simulink model "control_3quads_attached_Kumar"  (R2019a)
settings: Solver=FixedStepAuto  StartTime=0.0  StopTime=10  FixedStep=0.025  RelTol=1e-3  EnableMultiTasking=on
InitFcn:
  | global clientID;
  | clientID=-1;
  | 
  | global R_t;
  | global A_t;
  | global P_t;
  | global H;
  | global Q;
  | global N;
  | 
  | R_t=eye(3);
  | A_t=eye(3)*0;
  | P_t=eye(3)*0.001;
  | H=eye(3);
  | Q=eye(3);
  | N=eye(3);
undefined symbols (not defined in the file or in its folder): Angular, Linear, sigbuilder_block
libraries: robotlib x7, dspindex x3, simulink x1
settings Model: Creator=Kleber Cabral  LastModifiedBy=Kleber Cabral
settings DataIOCC: SaveFormat=Array  ReturnWorkspaceOutputs=off
settings OptimizationCC: LifeSpan=inf
settings DebuggingCC: SolverPrmCheckMsg=warning  SFUnexpectedBacktrackingDiag=warning  SFNoUnconditionalDefaultTransitionDiag=warning  ArithmeticOperatorsInVariantConditions=warning
settings HardwareCC: ProdBitPerPointer=32  ProdBitPerSizeT=32  ProdBitPerPtrDiffT=32  ProdLargestAtomicFloat=None  ProdIntDivRoundTo=Undefined  ProdEndianess=Unspecified  ProdWordSize=32  ProdHWDeviceType=32-bit Generic
settings ModelReferenceCC: PropagateSignalLabelsOutOfModel=off
settings SFSimCC: SimUseLocalCustomCode=off
settings RTWCC: RTWUseLocalCustomCode=off
settings CodeAppCC: StateflowObjectComments=on
settings GRTTargetCC: TargetLangStandard=C89/C90 (ANSI)  GeneratePreprocessorConditionals=Disable all
settings ConfigComp: CovMetricSettings=dw  CovHtmlReporting=on  CovSaveCumulativeToWorkspaceVar=on  CovSaveSingleToWorkspaceVar=on  CovExternalEMLEnable=off  CovSFcnEnable=off

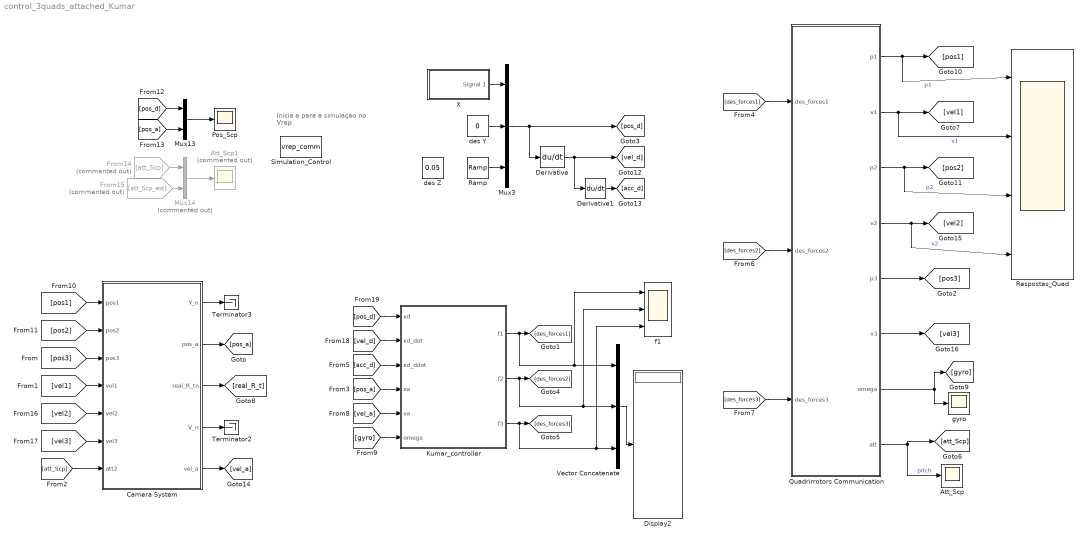
== system control_3quads_attached_Kumar ==
  note: Inicia e para a simulaçao no Vrep
  Att_Scp : Scope
  Att_Scp1 : Scope  Commented=on
  Camera System : Subsystem
  Derivative : Derivative
  Derivative1 : Derivative
  Display2 : Display
      settings: Decimation=3
  From14 : From  Commented=on  GotoTag=att_Scp
  From15 : From  Commented=on  GotoTag=att_Scp_est
  Kumar_controller : MATLAB Function  TreatAsAtomicUnit=on
  Mux13 : Mux  Inputs=2
  Mux14 : Mux  Commented=on  Inputs=2
  Mux3 : Mux  Inputs=3
  Pos_Scp : Scope
  Quadrirrotors Communication : Subsystem
  Ramp : simulink/Sources/Ramp  slope=0.05  start=1  InitialOutput=0
  Respostas_Quad : Scope  NumInputPorts=4
  Simulation_Control : S-Function  FunctionName=vrep_comm  SFunctionDeploymentMode=off  EnableBusSupport=off
  Terminator2 : Terminator
  Terminator3 : Terminator
  Vector Concatenate : Concatenate  NumInputs=3
  X : Subsystem  Tag=STV Subsys  LoadFcn=sigbuilder_block('load');  StartFcn=sigbuilder_block('start');  StopFcn=sigbuilder_block('stop');  ClipboardFcn=sigbuilder_block('clipboard');  mask(Sigbuilder block){tuvar=[0:10]}
      mask help: Simulink:masks:SigbuilderBlock_MD
      mask init:
      | if ~strcmp(get_param(bdroot(gcbh),'SimulationStatus'),'stopped') tuvar = sigbuilder_block('maskInit'); end
      settings: CopyFcn=sigbuilder_block('copy');  DeleteFcn=sigbuilder_block('delete');  ModelCloseFcn=sigbuilder_block('modelClose');  PreSaveFcn=sigbuilder_block('preSave');  PauseFcn=sigbuilder_block('pause');  ContinueFcn=sigbuilder_block('continue');  NameChangeFcn=sigbuilder_block('namechange');  OpenFcn=sigbuilder_block('open',[40.5 0 1393.5 802.5 ]);  CloseFcn=sigbuilder_block('close');
      mask Display: plot(0, 0, 100, 100,[2, 2, 32, 32, 2], [68, 8, 8, 68, 68],[32, 2], [38, 38], [32, 19, 2],[53, 60, 44], [32, 17, 17, 2],[16, 16, 31, 31]);txt = getActiveGroup(gcbh);text(2, 100, txt,'verticalAlignment', 'top');
  des Y : Constant  Value=0
  des Z : Constant  Value=0.05
  f1 : Scope  NumInputPorts=3
  gyro : Scope
  wires:
  Quadrirrotors Communication/1(p1) -> Respostas_Quad/1, [pos1]  "p1"
  des Y/1 -> Mux3/2
  [pos1] -> Camera System/1(pos1)
  [pos2] -> Camera System/2(pos2)
  [des_forces1] -> Quadrirrotors Communication/1(des_forces1)
  [des_forces2] -> Quadrirrotors Communication/2(des_forces2)
  Camera System/2(pos_a) -> [pos_a]
  [att_Scp] -> Camera System/7(att2)
  Mux3/1 -> Derivative/1, [pos_d]
  Mux13/1 -> Pos_Scp/1
  [pos_d] -> Mux13/1
  [pos_a] -> Mux13/2
  From14/1 -> Mux14/1
  From15/1 -> Mux14/2
  Mux14/1 -> Att_Scp1/1
  Camera System/3(real_R_tn) -> [real_R_t]
  Camera System/4(V_n) -> Terminator2/1
  X/1(Signal 1) -> Mux3/1
  Derivative1/1 -> [acc_d]
  Derivative/1 -> Derivative1/1, [vel_d]
  [acc_d] -> Kumar_controller/3(xd_ddot)
  [vel_d] -> Kumar_controller/2(xd_dot)
  [pos_d] -> Kumar_controller/1(xd)
  Quadrirrotors Communication/2(v1) -> Respostas_Quad/2, [vel1]  "v1"
  Quadrirrotors Communication/3(p2) -> Respostas_Quad/3, [pos2]  "p2"
  Quadrirrotors Communication/4(v2) -> Respostas_Quad/4, [vel2]  "v2"
  Quadrirrotors Communication/7(omega) -> [gyro], gyro/1
  [pos_a] -> Kumar_controller/4(xa)
  [gyro] -> Kumar_controller/6(omega)
  Camera System/5(vel_a) -> [vel_a]
  [vel_a] -> Kumar_controller/5(va)
  Camera System/1(Y_n) -> Terminator3/1
  Kumar_controller/1(f1) -> f1/1, Vector Concatenate/1, [des_forces1]
  Kumar_controller/2(f2) -> f1/2, Vector Concatenate/2, [des_forces2]
  Kumar_controller/3(f3) -> f1/3, Vector Concatenate/3, [des_forces3]
  Vector Concatenate/1 -> Display2/1
  [des_forces3] -> Quadrirrotors Communication/3(des_forces3)
  Quadrirrotors Communication/8(att) -> [att_Scp], Att_Scp/1  "pitch"
  Quadrirrotors Communication/5(p3) -> [pos3]
  Quadrirrotors Communication/6(v3) -> [vel3]
  [pos3] -> Camera System/3(pos3)
  [vel1] -> Camera System/4(vel1)
  [vel3] -> Camera System/6(vel3)
  [vel2] -> Camera System/5(vel2)
  Ramp/1 -> Mux3/3

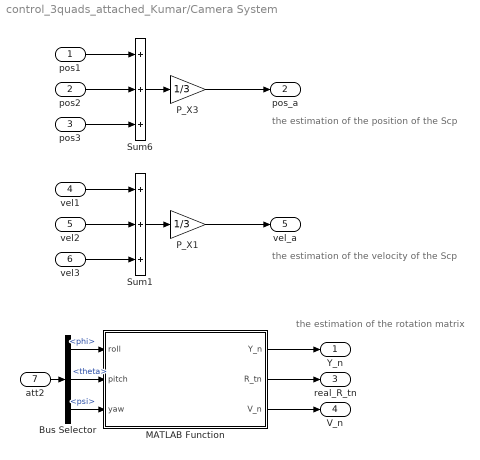
== system control_3quads_attached_Kumar/Camera System ==
  note: the estimation of the rotation matrix
  note: the estimation of the position of the Scp
  note: the estimation of the velocity of the Scp
  pos1 : Inport
  pos2 : Inport  Port=2
  pos3 : Inport  Port=3
  vel1 : Inport  Port=4
  vel2 : Inport  Port=5
  vel3 : Inport  Port=6
  att2 : Inport  Port=7
  Bus Selector : BusSelector  OutputSignals=phi,theta,psi
  MATLAB Function : MATLAB Function  TreatAsAtomicUnit=on
  P_X1 : Gain  Gain=1/3
  P_X3 : Gain  Gain=1/3
  Sum1 : Sum  Inputs=+++
  Sum6 : Sum  Inputs=+++
  Y_n : Outport
  pos_a : Outport  Port=2
  real_R_tn : Outport  Port=3
  V_n : Outport  Port=4
  vel_a : Outport  Port=5
  wires:
  pos1/1 -> Sum6/1
  pos2/1 -> Sum6/2
  Sum6/1 -> P_X3/1
  P_X3/1 -> pos_a/1
  att2/1 -> Bus Selector/1
  Bus Selector/3 -> MATLAB Function/3(yaw)  "<psi>"
  Bus Selector/2 -> MATLAB Function/2(pitch)  "<theta>"
  Bus Selector/1 -> MATLAB Function/1(roll)  "<phi>"
  MATLAB Function/1(Y_n) -> Y_n/1
  MATLAB Function/2(R_tn) -> real_R_tn/1
  MATLAB Function/3(V_n) -> V_n/1
  P_X1/1 -> vel_a/1
  pos3/1 -> Sum6/3
  vel1/1 -> Sum1/1
  vel2/1 -> Sum1/2
  vel3/1 -> Sum1/3
  Sum1/1 -> P_X1/1

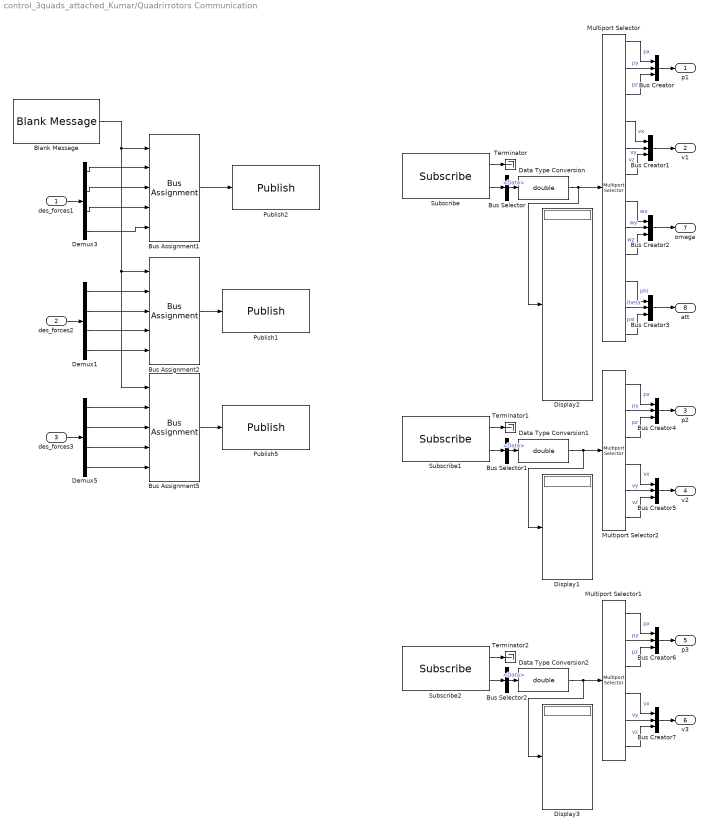
== system control_3quads_attached_Kumar/Quadrirrotors Communication ==
  des_forces1 : Inport
  des_forces2 : Inport  Port=2
  des_forces3 : Inport  Port=3
  Blank Message : robotlib/Blank Message  messageClass=Message  entityType=geometry_msgs/Twist  messageType=geometry_msgs/Twist  SampleTime=inf
      settings: SourceProductBaseCode=RO
  Bus Assignment1 : BusAssignment  DialogController=Simulink.DDGSource_BusAssignment  AssignedSignals=Linear.X,Linear.Y,Angular.X,Angular.Y
  Bus Assignment2 : BusAssignment  DialogController=Simulink.DDGSource_BusAssignment  AssignedSignals=Linear.X,Linear.Y,Angular.X,Angular.Y
  Bus Assignment5 : BusAssignment  DialogController=Simulink.DDGSource_BusAssignment  AssignedSignals=Linear.X,Linear.Y,Angular.X,Angular.Y
  Bus Creator{,1..7} (8 alike) : BusCreator  Inputs=3
  Bus Selector : BusSelector  OutputSignals=Data
  Bus Selector1 : BusSelector  OutputSignals=Data
  Bus Selector2 : BusSelector  OutputSignals=Data
  Data Type Conversion : DataTypeConversion  OutDataTypeStr=double
  Data Type Conversion1 : DataTypeConversion  OutDataTypeStr=double
  Data Type Conversion2 : DataTypeConversion  OutDataTypeStr=double
  Demux1 : Demux
  Demux3 : Demux
  Demux5 : Demux
  Display1 : Display
      settings: Decimation=3
  Display2 : Display
      settings: Decimation=3
  Display3 : Display
      settings: Decimation=3
  Multiport Selector : dspindex/Multiport Selector  rowsOrCols=Rows  idxCellArray={1,2,3,4,5,6,7,8,9,10,11,12}  idxErrMode=Clip Index
  Multiport Selector1 : dspindex/Multiport Selector  rowsOrCols=Rows  idxCellArray={1,2,3,4,5,6}  idxErrMode=Clip Index
  Multiport Selector2 : dspindex/Multiport Selector  rowsOrCols=Rows  idxCellArray={1,2,3,4,5,6}  idxErrMode=Clip Index
  Publish1 : robotlib/Publish  topicSource=Select from ROS network  topic=/motor_forces_1  messageType=geometry_msgs/Twist  messageQueueLength=105
      settings: SourceProductBaseCode=RO
  Publish2 : robotlib/Publish  topicSource=Select from ROS network  topic=/motor_forces_0  messageType=geometry_msgs/Twist  messageQueueLength=105
      settings: SourceProductBaseCode=RO
  Publish5 : robotlib/Publish  topicSource=Select from ROS network  topic=/motor_forces_2  messageType=geometry_msgs/Twist  messageQueueLength=105
      settings: SourceProductBaseCode=RO
  Subscribe : robotlib/Subscribe  topicSource=Select from ROS network  topic=/quadrotor_states_0  messageType=std_msgs/Float32MultiArray  sampleTime=-1  messageQueueLength=51
      settings: SourceProductBaseCode=RO
  Subscribe1 : robotlib/Subscribe  topicSource=Select from ROS network  topic=/quadrotor_states_1  messageType=std_msgs/Float32MultiArray  sampleTime=-1  messageQueueLength=51
      settings: SourceProductBaseCode=RO
  Subscribe2 : robotlib/Subscribe  topicSource=Select from ROS network  topic=/quadrotor_states_1  messageType=std_msgs/Float32MultiArray  sampleTime=-1  messageQueueLength=51
      settings: SourceProductBaseCode=RO
  Terminator : Terminator
  Terminator1 : Terminator
  Terminator2 : Terminator
  p1 : Outport
  v1 : Outport  Port=2
  p2 : Outport  Port=3
  v2 : Outport  Port=4
  p3 : Outport  Port=5
  v3 : Outport  Port=6
  omega : Outport  Port=7
  att : Outport  Port=8
  wires:
  Subscribe/1 -> Terminator/1
  Subscribe/2 -> Bus Selector/1
  Data Type Conversion/1 -> Display2/1, Multiport Selector/1
  Bus Selector/1 -> Data Type Conversion/1  "<Data>"
  Bus Assignment1/1 -> Publish2/1
  Bus Assignment2/1 -> Publish1/1
  Subscribe1/1 -> Terminator1/1
  Subscribe1/2 -> Bus Selector1/1
  Data Type Conversion1/1 -> Display1/1, Multiport Selector2/1
  Bus Selector1/1 -> Data Type Conversion1/1  "<Data>"
  Multiport Selector2/1 -> Bus Creator4/1  "px"
  Multiport Selector2/2 -> Bus Creator4/2  "py"
  Multiport Selector2/3 -> Bus Creator4/3  "pz"
  Multiport Selector2/4 -> Bus Creator5/1  "vx"
  Multiport Selector2/5 -> Bus Creator5/2  "vy"
  Multiport Selector2/6 -> Bus Creator5/3  "vz"
  des_forces1/1 -> Demux3/1
  Demux3/1 -> Bus Assignment1/2
  Demux3/2 -> Bus Assignment1/3
  Demux3/3 -> Bus Assignment1/4
  des_forces2/1 -> Demux1/1
  Multiport Selector/10 -> Bus Creator3/1  "phi"
  Multiport Selector/11 -> Bus Creator3/2  "theta"
  Multiport Selector/12 -> Bus Creator3/3  "psi"
  Bus Creator/1 -> p1/1
  Multiport Selector/2 -> Bus Creator/2  "py"
  Multiport Selector/1 -> Bus Creator/1  "px"
  Multiport Selector/3 -> Bus Creator/3  "pz"
  Multiport Selector/5 -> Bus Creator1/2  "vy"
  Multiport Selector/4 -> Bus Creator1/1  "vx"
  Multiport Selector/6 -> Bus Creator1/3  "vz"
  Bus Creator1/1 -> v1/1
  Multiport Selector/8 -> Bus Creator2/2  "wy"
  Multiport Selector/7 -> Bus Creator2/1  "wx"
  Multiport Selector/9 -> Bus Creator2/3  "wz"
  Bus Creator2/1 -> omega/1
  Bus Creator3/1 -> att/1
  Bus Creator4/1 -> p2/1
  Bus Creator5/1 -> v2/1
  Bus Creator7/1 -> v3/1
  Bus Creator6/1 -> p3/1
  Multiport Selector1/6 -> Bus Creator7/3  "vz"
  Multiport Selector1/5 -> Bus Creator7/2  "vy"
  Multiport Selector1/4 -> Bus Creator7/1  "vx"
  Multiport Selector1/3 -> Bus Creator6/3  "pz"
  Multiport Selector1/2 -> Bus Creator6/2  "py"
  Multiport Selector1/1 -> Bus Creator6/1  "px"
  Bus Selector2/1 -> Data Type Conversion2/1  "<Data>"
  Data Type Conversion2/1 -> Multiport Selector1/1, Display3/1
  Subscribe2/2 -> Bus Selector2/1
  Subscribe2/1 -> Terminator2/1
  Blank Message/1 -> Bus Assignment5/1, Bus Assignment2/1, Bus Assignment1/1
  Demux1/1 -> Bus Assignment2/2
  Demux1/2 -> Bus Assignment2/3
  Demux1/3 -> Bus Assignment2/4
  Demux1/4 -> Bus Assignment2/5
  Demux3/4 -> Bus Assignment1/5
  Demux5/4 -> Bus Assignment5/5
  Demux5/3 -> Bus Assignment5/4
  Demux5/2 -> Bus Assignment5/3
  Demux5/1 -> Bus Assignment5/2
  des_forces3/1 -> Demux5/1
  Bus Assignment5/1 -> Publish5/1

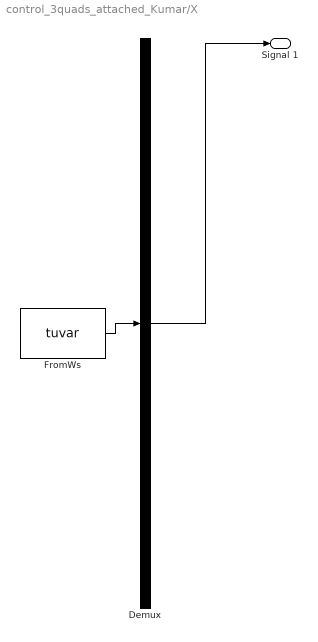
== system control_3quads_attached_Kumar/X ==
  Demux : Demux  Tag=STV Demux  Outputs=1
  FromWs : FromWorkspace  Tag=STV FromWs  VariableName=tuvar  SampleTime=0
      SigBuilderData=|
      | common.afterFinalStr = 'Extrapolate'
      | common.sampleTime = 0
      | dataSet.timeRange = [0 60]
      | dataSet.name = 'Group 1'
      | sbobj.Groups.Name = 'Group 1'
      | sbobj.Groups.Signals.Name = 'Signal 1'
      | sbobj.Groups.Signals.XData = [0 20 20.3 20.5 29.55 29.75 30 40 40.2 40.35 49.55 49.75 50 60]
      | sbobj.Groups.Signals.YData = [0 0 0.008 0.018 0.98 0.992 1 1 0.994 0.986 0.02 0.008 0 0]
      | sbobj.Groups.TimeRange = [0 60]
  Signal 1 : Outport  Tag=STV Outport
  wires:
  Demux/1 -> Signal 1/1
  FromWs/1 -> Demux/1

== matlab function control_3quads_attached_Kumar/Kumar_controller ==
  data: xd input; f1 output; xd_dot input; xd_ddot input; xa input; va input; omega input; f2 output; f3 output
function [f1,f2,f3]  = Kumar_controller(xd,xd_dot,xd_ddot,xa,va,omega)
%cooperative transportation controller from Vijay kumar

dt=0.025;

%part position
x_1 = -0.135;%distance from center of compound part
y_1 = 0;%distance from center of compound part

%part position
x_2 = 0;%distance from center of compound part
y_2 = 0;%distance from center of compound part

x_3 = 0.135;%distance from center of compound part
y_3 = 0;%distance from center of compound part

psi_1=0;

A_1 =[ 1 0 0 0;
       y_1 cos(psi_1) -sin(psi_1) 0;
       -x_1 sin(psi_1)  cos(psi_1) 0;
       0 0 0 1];
   
A_2 =[ 1 0 0 0;
   y_2 cos(0) -sin(0) 0;
   -x_2 sin(0)  cos(0) 0;
   0 0 0 1];
   
A_3 =[ 1 0 0 0;
   y_3 cos(0) -sin(0) 0;
   -x_3 sin(0)  cos(0) 0;
   0 0 0 1];

arm_length=0.042;
l=(sqrt(2)/2) * arm_length;
c=0.001;% force to torque relationship in the propeller
P=[1,1,1,1; l,-l,-l,l; -l,-l,l,l; c,-c,c,-c];

K=[A_1*P A_2*P A_3*P];

e3=[0;0;1]; %inertial z vector

J=diag([0.001*3;0.001;0.01]); %Inertia matrix

W = eye(12); %importance of each motor in the control

%Gains
kx=1;
kv=1;
kR=0.1;
kO=0.1;
m=0.165;
g=9.82;
f=zeros(12,1);

% computed attitude Rc(t) ? SO(3) and 
% computed angular velocity Oc ? R3

R=eye(3);

% omega angular velocity comes from sensors vrep
% R = [b1,b2,b3] attitude from body vectors

%computing errors

ex = xa - xd;
ev = va - xd_dot;
omega_hat=skew_sym_3(omega);

% Compound part control, position and attitude
%Find the desired moments and thrust

%compute the desired force first
Fdes = m*g*e3 + m*xd_ddot -kx*ex - kv*ev ;
T = dot(Fdes,R*e3)

%use the desired force vector to find the desired rotation
zbdes= Fdes/norm(Fdes);
xcdes=[1;0;0];
ybdes=cross(zbdes,xcdes)/norm(cross(zbdes,xcdes));
xbdes=cross(ybdes,zbdes);
Rdes=[xbdes,ybdes,zbdes];

Rdes_dot=Rdes*skew_sym_3(omega);
omegades = vee_map(Rdes'*Rdes_dot);
omegades_dot = (vee_map(Rdes'*Rdes_dot)-omegades)/ dt;

%compute the errors in rotation
eO= omega - R' * Rdes * omegades;
eR= 0.5*vee_map(Rdes' * R - R' * Rdes);
M =  - kR*eR - kO*eO + cross(omega,J*omega) - J*(omega_hat*R'*Rdes*omegades - R'*Rdes*omegades_dot);

u=[T;M];

%given desired control inputs, find motor speeds
Kcross=inv(W) * K' * inv( K * inv(W) * K');
f=Kcross*u;
f=max(min(f,0.5),0);
f1=f(1:4);
f2=f(5:8);
f3=f(9:12);
end

== matlab function control_3quads_attached_Kumar/Camera System/MATLAB Function ==
  data: roll input; Y_n output; pitch input; yaw input; R_tn output; V_n output
function [Y_n,R_tn,V_n] = EulerAng2RotMat(roll, pitch, yaw)
% a=deg2rad(0);
% b=deg2rad(0);
% c=deg2rad(45);

a=roll;
b=pitch;
c=yaw;

sa=sin(a);ca=cos(a);
sb=sin(b);cb=cos(b);
sc=sin(c);cc=cos(c);
R_tn=[ cc*cb cc*sb*sa-sc*ca cc*sb*ca+sc*sa 
    sc*cb sc*sb*sa+cc*ca sc*sb*ca-cc*sa 
    -sb       cb*sa           cb*ca     ];

%noise of about 1 deg of rotation in each axis
a=deg2rad(randn);
b=deg2rad(randn);
c=deg2rad(randn);
sa=sin(a);ca=cos(a);
sb=sin(b);cb=cos(b);
sc=sin(c);cc=cos(c);
V_n=[ cc*cb cc*sb*sa-sc*ca cc*sb*ca+sc*sa 
    sc*cb sc*sb*sa+cc*ca sc*sb*ca-cc*sa 
    -sb       cb*sa           cb*ca     ];

Y_n = R_tn * V_n;

%R = R *(eye(3)+0.001*randn(3,3));
end
